simulink model "sawtooth_neuroFuzzy"  (R2017b)
settings: Solver=FixedStepAuto  StartTime=0.0  StopTime=500.0  RelTol=1e-3  EnableMultiTasking=on
libraries: fuzblock x1
settings Model: Creator=metalhead  LastModifiedBy=root
settings DataIOCC: LimitDataPoints=on
settings OptimizationCC: LifeSpan=inf
settings DebuggingCC: AllowSymbolicDim=off  SFUnexpectedBacktrackingDiag=warning  SFNoUnconditionalDefaultTransitionDiag=warning  SFExecutionAtInitializationDiag=none
settings ModelReferenceCC: PropagateSignalLabelsOutOfModel=off
settings CodeAppCC: StateflowObjectComments=on
settings GRTTargetCC: TargetLangStandard=C89/C90 (ANSI)
settings ConfigComp: CovMetricSettings=dw  CovHtmlReporting=on  CovSaveCumulativeToWorkspaceVar=on  CovSaveSingleToWorkspaceVar=on  CovExternalEMLEnable=off

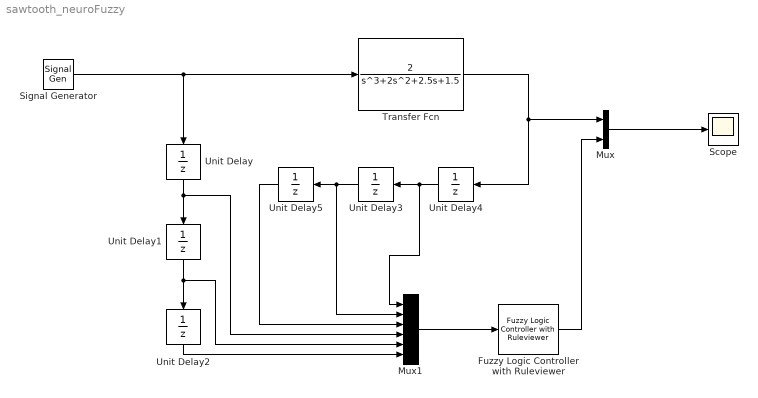
== system sawtooth_neuroFuzzy ==
  Fuzzy Logic Controller with Ruleviewer : fuzblock/Fuzzy Logic  Controller  with Ruleviewer  fismatrix=controller  Ts=1
  Mux : Mux  Inputs=2
  Mux1 : Mux  Inputs=6
  Scope : Scope
  Signal Generator : SignalGenerator  WaveForm=sawtooth  Frequency=0.1  Units=rad/sec
  Transfer Fcn : TransferFcn  Numerator=[2]  Denominator=[1 2 2.5 1.5]
  Unit Delay{,1..5} (6 alike) : UnitDelay  SampleTime=-1
  wires:
  Signal Generator/1 -> Transfer Fcn/1, Unit Delay/1
  Unit Delay/1 -> Mux1/4, Unit Delay1/1
  Unit Delay1/1 -> Mux1/5, Unit Delay2/1
  Transfer Fcn/1 -> Mux/1, Unit Delay4/1
  Unit Delay4/1 -> Mux1/1, Unit Delay3/1
  Unit Delay3/1 -> Mux1/2, Unit Delay5/1
  Unit Delay5/1 -> Mux1/3
  Unit Delay2/1 -> Mux1/6
  Mux1/1 -> Fuzzy Logic Controller with Ruleviewer/1
  Fuzzy Logic Controller with Ruleviewer/1 -> Mux/2
  Mux/1 -> Scope/1
